simulink model "MovRotacionalSimulink"  (R2024b)
settings: Solver=VariableStepAuto  StartTime=0.0  StopTime=10.0  MaxStep=0.01  RelTol=1e-3
InitFcn:
  | m = 10;
  | r = 0.05;
  | k = 100;
settings Model: Creator=newju  LastModifiedBy=newju

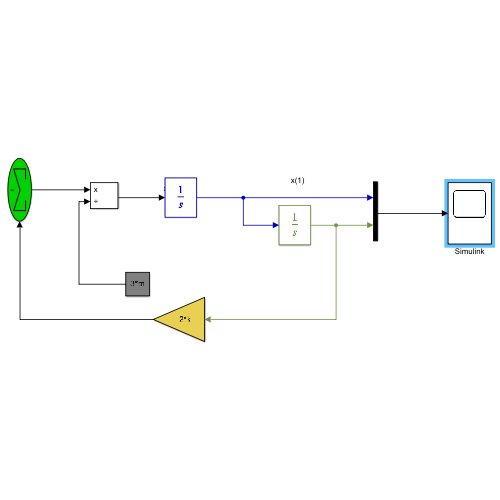
[thumbnail: Simulink's stored preview of the top-level diagram]
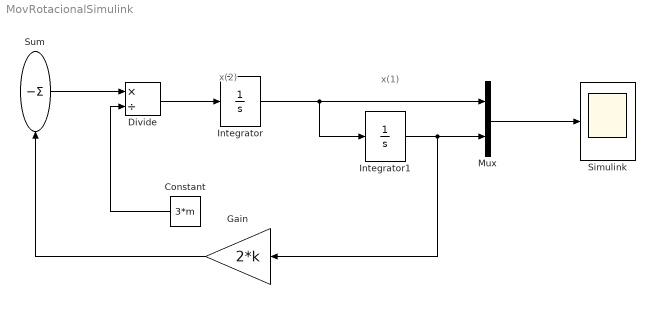
== system MovRotacionalSimulink ==
  note: x(2)
  note: x(1)
  Constant : Constant  Value=3*m
  Divide : Product  Inputs=*/
  Gain : Gain  Gain=2*k
  Integrator : Integrator  InitialCondition=2
  Integrator1 : Integrator
  Mux : Mux  Inputs=2
  Simulink : Scope
  Sum : Sum  Inputs=|-
  wires:
  Mux/1 -> Simulink/1
  Integrator1/1 -> Gain/1, Mux/2
  Integrator/1 -> Integrator1/1, Mux/1
  Sum/1 -> Divide/1
  Gain/1 -> Sum/1
  Divide/1 -> Integrator/1
  Constant/1 -> Divide/2
